simulink model "FINALCODE"  (R2018a)
settings: Solver=VariableStepAuto  StartTime=0.0  StopTime=10.0  RelTol=1e-3
libraries: commcnvcod2 x2, dspxfrm3 x2, commblkintrlv2 x2, commdigbbndam3 x2, commchan3 x1, commrandsrc3 x1, commsink2 x1
settings Model: Creator=Farhath  LastModifiedBy=YMTS0534

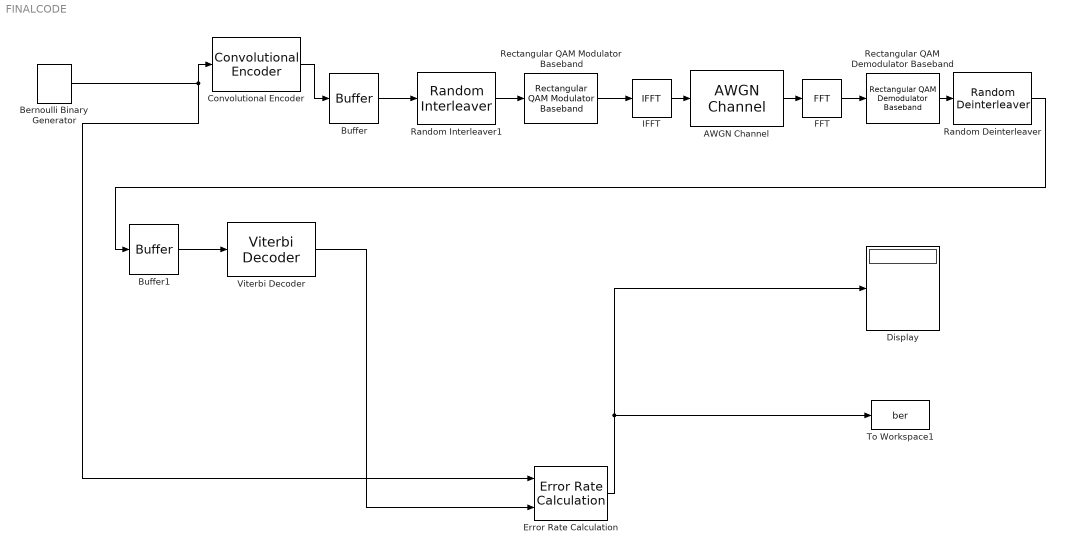
== system FINALCODE ==
  AWGN Channel : commchan3/AWGN Channel  InputProcessing=Columns as channels (frame based)  seed=67  noiseMode="Signal to noise ratio  (Eb/No)"  EbNodB=10  EsNodB=10  SNRdB=10  bitsPerSym=1  Ps=1  Tsym=1  variance=1
  Bernoulli Binary Generator : commrandsrc3/Bernoulli Binary Generator  ProbabilityOfZero=0.5  SeedSource=Parameter  Seed=[10^9]  SampleTime=1  SamplesPerFrame=1  OutputDataType=double  SimulateUsing=Interpreted execution
  Buffer : Buffer  N=50  OutputFrames=off
  Buffer1 : Buffer  N=50  OutputFrames=off
  Convolutional Encoder : commcnvcod2/Convolutional Encoder  trellis=poly2trellis(7, [171 133])  opMode=Continuous  DelayedResetAction=off  hasIniStPort=off  hasFinStPort=off  usePuncVector=off  punctureVector=[1; 1; 0; 1; 0; 1]  reset=Unused parameter value
      settings: SourceProductName=Communications System Toolbox  SourceProductBaseCode=CM
  Display : Display
  Error Rate Calculation : commsink2/Error Rate Calculation  N=0  st_delay=0  cp_mode=Entire frame  subframe=[35]  PMode=Port  WsName=ErrorVec  RsMode2=off  stop=on  numErr=100  maxBits=1e8
  FFT : dspxfrm3/FFT  FFTImplementation=Auto  CompMethod=Table lookup  TableOpt=NEW  TableOptActive=Speed  BitRevOrder=off  Normalize=off  InheritFFTLength=on  FFTLength=64  WrapInput=on  roundingMode=Floor  overflowMode=off  firstCoeffDataTypeStr=Inherit: Same word length as input  firstCoeffLastDataTypeStr=Inherit: Same word length as input  outputMin=[]  outputMax=[]
  IFFT : dspxfrm3/IFFT  FFTImplementation=Auto  CompMethod=Table lookup  TableOpt=NEW  TableOptActive=Speed  BitRevOrder=off  cs_in=off  Normalize=on  InheritFFTLength=on  FFTLength=64  WrapInput=on  mode=Complex  outSamplingMode=Sample based  roundingMode=Floor  overflowMode=off  firstCoeffDataTypeStr=Inherit: Same word length as input  firstCoeffLastDataTypeStr=Inherit: Same word length as input  outputMin=[]  outputMax=[]
      settings: SourceProductName=DSP System Toolbox
  Random Deinterleaver : commblkintrlv2/Random Deinterleaver  N=50  seed=12345
      settings: SourceProductName=Communications System Toolbox  SourceProductBaseCode=CM
  Random Interleaver1 : commblkintrlv2/Random Interleaver  N=50  seed=12345
      settings: SourceProductName=Communications System Toolbox  SourceProductBaseCode=CM
  Rectangular QAM Demodulator Baseband : commdigbbndam3/Rectangular QAM Demodulator Baseband  M=64  OutType=Integer  DecType=Hard decision  VarSource=Dialog  Variance=1  Dec=Gray  Mapping=[0:15]  PowType=Min. distance between symbols  MinDist=2  AvgPow=1  PeakPow=1  Ph=0  outDtype1=Inherit via internal rule  outDtype2=Inherit via internal rule  derotateFactorWordLen=16  derotateFactorDataTypeStr=Inherit: Same word length as input  derotateFactorLastDataTypeStr=Inherit: Same word length as input  denormFactorWordLen=16  denormFactorDataTypeStr=Inherit: Same word length as input  denormFactorLastDataTypeStr=Inherit: Same word length as input  prodOutWordLen=32  prodOutOverflowMode=Wrap  prodOutRoundingMode=Floor  prodOutOvFlMode=off  prodOutOvFlModeLastStrValue=off  sumWordLen=32
  Rectangular QAM Modulator Baseband : commdigbbndam3/Rectangular QAM Modulator Baseband  M=64  InType=Integer  Enc=Gray  Mapping=[0:15]  PowType=Min. distance between symbols  MinDist=2  AvgPow=1  PeakPow=1  Ph=0  outDtype=double  outWordLen=16  outUDDataType=sfix(16)  outFracLenMode=Best precision  outFracLen=15  outDataTypeStr=double  outLastDataTypeStr=double
  To Workspace1 : ToWorkspace  VariableName=ber  SampleTime=-1
      settings: Save2DSignal=2-D array (concatenate along first dimension)
  Viterbi Decoder : commcnvcod2/Viterbi Decoder  trellis=poly2trellis(7, [171 133])  isPunctured=off  punctureVector=[1; 1; 0; 1; 0; 1]  erasures=off  dectype=Unquantized  nsdecb=4  runSigValErrCheck=off  tbdepth=34  opmode=Continuous  reset=off  delayedResetAction=off  smWordLength=16  outDataType=Inherit via internal rule
      settings: SourceProductName=Communications System Toolbox  SourceProductBaseCode=CM
  wires:
  Convolutional Encoder/1 -> Buffer/1
  Buffer/1 -> Random Interleaver1/1
  Random Interleaver1/1 -> Rectangular QAM Modulator Baseband/1
  Rectangular QAM Modulator Baseband/1 -> IFFT/1
  IFFT/1 -> AWGN Channel/1
  AWGN Channel/1 -> FFT/1
  FFT/1 -> Rectangular QAM Demodulator Baseband/1
  Rectangular QAM Demodulator Baseband/1 -> Random Deinterleaver/1
  Random Deinterleaver/1 -> Buffer1/1
  Buffer1/1 -> Viterbi Decoder/1
  Bernoulli Binary Generator/1 -> Error Rate Calculation/1, Convolutional Encoder/1
  Viterbi Decoder/1 -> Error Rate Calculation/2
  Error Rate Calculation/1 -> Display/1, To Workspace1/1
